simulink model "RC_model"  (Simulink 7.0)
settings: Solver=ode4  StartTime=0.0  StopTime=1  FixedStep=0.01  MaxStep=0.25  RelTol=1e-3
settings Model: Creator=adminus  LastModifiedBy=adminus

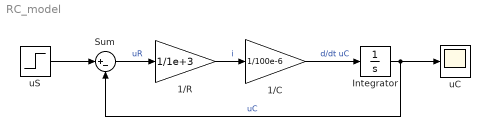
== system RC_model ==
  1/C : Gain  Gain=1/100e-6  ParameterDataType=sfix(16)  ParameterScaling=2^0  OutDataType=sfix(16)  OutScaling=2^0
  1/R : Gain  Gain=1/1e+3  ParameterDataType=sfix(16)  ParameterScaling=2^0  OutDataType=sfix(16)  OutScaling=2^0
  Integrator : Integrator
  Sum : Sum  Inputs=|+-  OutDataType=sfix(16)  OutScaling=2^0
  uC : Scope
  uS : Step  Time=0  SampleTime=0
  wires:
  uS/1 -> Sum/1
  Sum/1 -> 1/R/1  "uR"
  1/R/1 -> 1/C/1  "i"
  1/C/1 -> Integrator/1  "d/dt uC"
  Integrator/1 -> uC/1, Sum/2  "uC"
